simulink model "Motor_PID_discreto"  (R2017b)
settings: Solver=VariableStepAuto  StartTime=0.0  StopTime=3  RelTol=1e-3
values from neighbouring files (symbols this model uses):
  Bm = 0    [TP1_MOTOR_1.m]    (also in TP1_MOTOR_3.m = 0.01)
  J = 5e-9    (= 5e-09)    [TP1_MOTOR_1.m]    (also in TP1_MOTOR_3.m = 3e-05)
  Ki = 6.49e-3    (= 0.00649)    [TP1_MOTOR_1.m]    (also in TP1_MOTOR_3.m = num(3))
  Km = 6.53e-3    (= 0.00653)    [TP1_MOTOR_1.m]    (also in TP1_MOTOR_3.m = (den(3)-Ra*Bm)/Ki)
  Laa = 366e-6    (= 0.000366)    [TP1_MOTOR_1.m]    (also in TP1_MOTOR_3.m = den(1)/J)
  num = num/12    [TP1_MOTOR_3.m]
  numi = numi/0.075    [TP1_MOTOR_3.m]
  Ra = 55.6    [TP1_MOTOR_1.m]    (also in TP1_MOTOR_3.m = (den(2)-Laa*Bm)/J)
undefined symbols (not defined in the file or in its folder): den, deni
libraries: simulink x2
settings Model: Creator=feder  LastModifiedBy=feder

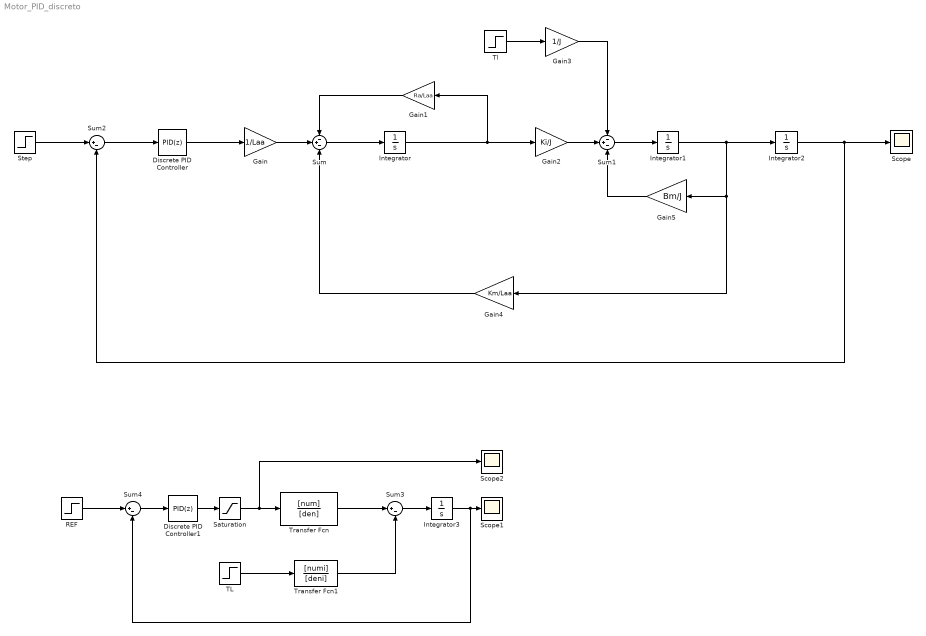
== system Motor_PID_discreto ==
  Discrete PID Controller : simulink/Continuous/PID Controller  Controller=PID  TimeDomain=Discrete-time  SampleTime=0.00001  IntegratorMethod=Forward Euler  FilterMethod=Forward Euler  Form=Parallel  UseFilter=off  ControllerParametersSource=internal  P=30  I=100  D=0.1  N=100  InitialConditionSource=internal  InitialConditionForIntegrator=0  InitialConditionForFilter=0  ExternalReset=none  LimitOutput=off  UpperSaturationLimit=inf  LowerSaturationLimit=-inf  LinearizeAsGain=off  AntiWindupMode=none  Kb=1  TrackingMode=off  Kt=1  PParamMin=[]  PParamMax=[]  IParamMin=[]  IParamMax=[]  DParamMin=[]  DParamMax=[]  NParamMin=[]  NParamMax=[]  KbParamMin=[]  KbParamMax=[]  KtParamMin=[]  KtParamMax=[]  POutMin=[]  POutMax=[]  IOutMin=[]  IOutMax=[]  DOutMin=[]  DOutMax=[]  NOutMin=[]  NOutMax=[]  KbOutMin=[]  KbOutMax=[]  KtOutMin=[]  KtOutMax=[]  IntegratorOutMin=[]  IntegratorOutMax=[]  FilterOutMin=[]  FilterOutMax=[]  SumOutMin=[]  SumOutMax=[]  SumI1OutMin=[]  SumI1OutMax=[]  SumI2OutMin=[]  SumI2OutMax=[]  SumI3OutMin=[]  SumI3OutMax=[]  SumDOutMin=[]  SumDOutMax=[]  SaturationOutMin=[]  SaturationOutMax=[]  IntegratorContinuousStateAttributes=''  IntegratorStateMustResolveToSignalObject=off  IntegratorRTWStateStorageClass=Auto  FilterContinuousStateAttributes=''  FilterStateMustResolveToSignalObject=off  FilterRTWStateStorageClass=Auto  DifferentiatorICPrevScaledInput=0  DifferentiatorOutMin=[]  DifferentiatorOutMax=[]  InitialConditionSetting=State (most efficient)  FilterDiffOutCoefMin=[]  FilterDiffOutCoefMax=[]  SumDenOutMin=[]  SumDenOutMax=[]  SumNumOutMin=[]  SumNumOutMax=[]  ReciprocalOutMin=[]  ReciprocalOutMax=[]  DivideOutMin=[]  DivideOutMax=[]  TunerSelectOption=Transfer Function Based (PID Tuner App)
  Discrete PID Controller1 : simulink/Continuous/PID Controller  Controller=PID  TimeDomain=Discrete-time  SampleTime=0.00001  IntegratorMethod=Forward Euler  FilterMethod=Forward Euler  Form=Parallel  UseFilter=off  ControllerParametersSource=internal  P=30  I=100  D=0.1  N=100  InitialConditionSource=internal  InitialConditionForIntegrator=0  InitialConditionForFilter=0  ExternalReset=none  LimitOutput=off  UpperSaturationLimit=inf  LowerSaturationLimit=-inf  LinearizeAsGain=off  AntiWindupMode=none  Kb=1  TrackingMode=off  Kt=1  PParamMin=[]  PParamMax=[]  IParamMin=[]  IParamMax=[]  DParamMin=[]  DParamMax=[]  NParamMin=[]  NParamMax=[]  KbParamMin=[]  KbParamMax=[]  KtParamMin=[]  KtParamMax=[]  POutMin=[]  POutMax=[]  IOutMin=[]  IOutMax=[]  DOutMin=[]  DOutMax=[]  NOutMin=[]  NOutMax=[]  KbOutMin=[]  KbOutMax=[]  KtOutMin=[]  KtOutMax=[]  IntegratorOutMin=[]  IntegratorOutMax=[]  FilterOutMin=[]  FilterOutMax=[]  SumOutMin=[]  SumOutMax=[]  SumI1OutMin=[]  SumI1OutMax=[]  SumI2OutMin=[]  SumI2OutMax=[]  SumI3OutMin=[]  SumI3OutMax=[]  SumDOutMin=[]  SumDOutMax=[]  SaturationOutMin=[]  SaturationOutMax=[]  IntegratorContinuousStateAttributes=''  IntegratorStateMustResolveToSignalObject=off  IntegratorRTWStateStorageClass=Auto  FilterContinuousStateAttributes=''  FilterStateMustResolveToSignalObject=off  FilterRTWStateStorageClass=Auto  DifferentiatorICPrevScaledInput=0  DifferentiatorOutMin=[]  DifferentiatorOutMax=[]  InitialConditionSetting=State (most efficient)  FilterDiffOutCoefMin=[]  FilterDiffOutCoefMax=[]  SumDenOutMin=[]  SumDenOutMax=[]  SumNumOutMin=[]  SumNumOutMax=[]  ReciprocalOutMin=[]  ReciprocalOutMax=[]  DivideOutMin=[]  DivideOutMax=[]  TunerSelectOption=Transfer Function Based (PID Tuner App)
  Gain : Gain  Gain=1/Laa
  Gain1 : Gain  Gain=Ra/Laa
  Gain2 : Gain  Gain=Ki/J
  Gain3 : Gain  Gain=1/J
  Gain4 : Gain  Gain=Km/Laa
  Gain5 : Gain  Gain=Bm/J
  Integrator{,1..3} (4 alike) : Integrator
  REF : Step  Time=0.02  SampleTime=0
  Saturation : Saturate  UpperLimit=12  LowerLimit=-12
  Scope : Scope
  Scope1 : Scope
  Scope2 : Scope
  Step : Step  Time=0.01  SampleTime=0
  Sum : Sum  Inputs=-+-
  Sum1 : Sum  Inputs=-+-
  Sum2 : Sum  Inputs=|+-
  Sum3 : Sum  Inputs=|+-
  Sum4 : Sum  Inputs=|+-
  TL : Step  Time=0.5  After=0.075  SampleTime=0
  "Tl " : Step  Time=0.7  After=0.007  SampleTime=0
  Transfer Fcn : TransferFcn  Numerator=[num]  Denominator=[den]
  Transfer Fcn1 : TransferFcn  Numerator=[numi]  Denominator=[deni]
  wires:
  Gain1/1 -> Sum/1
  Gain/1 -> Sum/2
  Sum/1 -> Integrator/1
  Integrator/1 -> Gain2/1, Gain1/1
  Sum1/1 -> Integrator1/1
  Integrator1/1 -> Integrator2/1, Gain5/1, Gain4/1
  Gain2/1 -> Sum1/2
  Gain3/1 -> Sum1/1
  "Tl "/1 -> Gain3/1
  Gain4/1 -> Sum/3
  Gain5/1 -> Sum1/3
  Integrator2/1 -> Scope/1, Sum2/2
  Step/1 -> Sum2/1
  Discrete PID Controller/1 -> Gain/1
  Sum2/1 -> Discrete PID Controller/1
  Transfer Fcn/1 -> Sum3/1
  TL/1 -> Transfer Fcn1/1
  Transfer Fcn1/1 -> Sum3/2
  Sum3/1 -> Integrator3/1
  Sum4/1 -> Discrete PID Controller1/1
  Integrator3/1 -> Sum4/2, Scope1/1
  REF/1 -> Sum4/1
  Discrete PID Controller1/1 -> Saturation/1
  Saturation/1 -> Scope2/1, Transfer Fcn/1
